simulink model "BatterySimulationCCCVwithFunction"  (R2018b)
settings: Solver=FixedStepAuto  StartTime=0.0  StopTime=2  FixedStep=0.01  MaxStep=0.01  MinStep=0.01  RelTol=1e-3
settings Model: Creator=GRosp  LastModifiedBy=GRosp

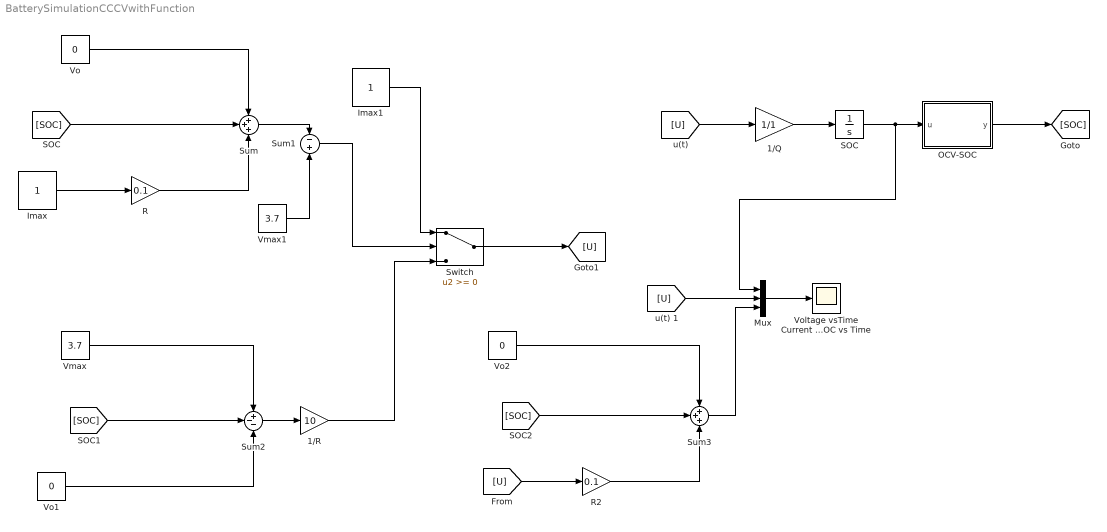
== system BatterySimulationCCCVwithFunction ==
  1/Q : Gain  Gain=1/1
  "1/R " : Gain  Gain=10
  Imax : Constant
  Imax1 : Constant
  Mux : Mux  Inputs=3
  OCV-SOC : MATLAB Function  TreatAsAtomicUnit=on
  R : Gain  Gain=0.1
  R2 : Gain  Gain=0.1
  "SOC " : Integrator
  Sum : Sum  Inputs=+++
  Sum1 : Sum  Inputs=-+
  Sum2 : Sum  Inputs=+--
  Sum3 : Sum  Inputs=+++
  Switch : Switch
  Vmax : Constant  Value=3.7
  "Vmax1 " : Constant  Value=3.7
  Vo : Constant  Value=0
  Vo1 : Constant  Value=0
  Vo2 : Constant  Value=0
  Voltage vsTime Current vs Time SOC vs Time : Scope
  wires:
  Vo/1 -> Sum/1
  1/Q/1 -> "SOC "/1
  [U] -> 1/Q/1
  Imax/1 -> R/1
  R/1 -> Sum/3
  Imax1/1 -> Switch/1
  Sum/1 -> Sum1/1
  "Vmax1 "/1 -> Sum1/2
  Sum1/1 -> Switch/2
  Switch/1 -> [U]
  Vmax/1 -> Sum2/1
  R2/1 -> Sum3/3
  Vo2/1 -> Sum3/1
  Sum2/1 -> "1/R "/1
  "1/R "/1 -> Switch/3
  Vo1/1 -> Sum2/3
  [U] -> R2/1
  Mux/1 -> Voltage vsTime Current vs Time SOC vs Time/1
  [SOC] -> Sum2/2
  [SOC] -> Sum/2
  "SOC "/1 -> Mux/1, OCV-SOC/1(u)
  [U] -> Mux/2
  Sum3/1 -> Mux/3
  OCV-SOC/1(y) -> [SOC]
  [SOC] -> Sum3/2

== matlab function BatterySimulationCCCVwithFunction/OCV-SOC ==
  data: u input; y output
function y = fcn(u)
y = 2.6+2.35*u-3.75*u^2+2.5*u^3;
